simulink model "BLDCmotor_controll"  (R2015b)
settings: Solver=VariableStepAuto  StartTime=0.0  StopTime=10.0  RelTol=1e-3
settings Model: Creator=shangwei  LastModifiedBy=root

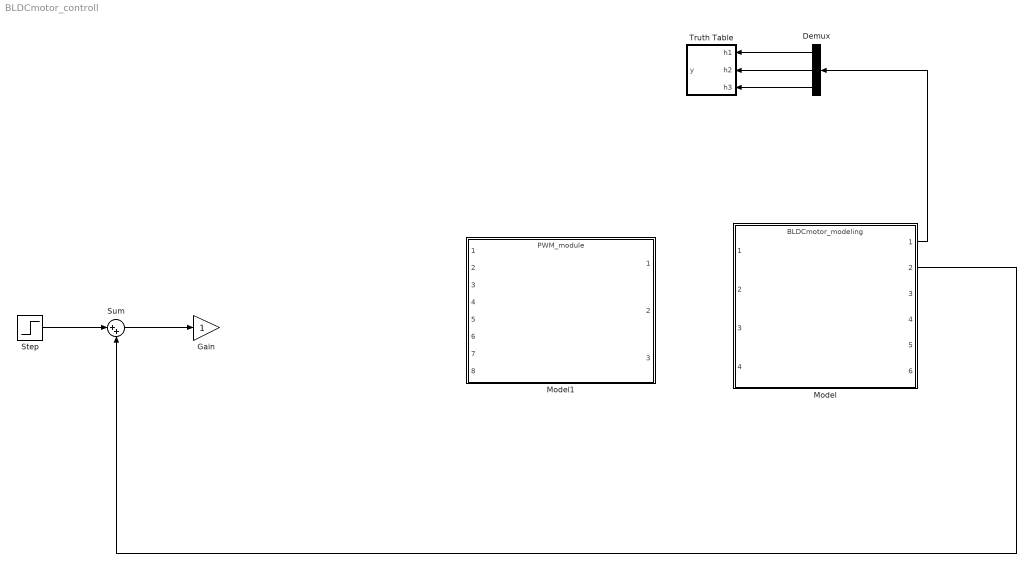
== system BLDCmotor_controll ==
  Demux : Demux  Outputs=3
  Gain : Gain
  Model : ModelReference  ModelNameDialog=BLDCmotor_modeling.slx  SimulationMode=Normal  ModelReferenceVersion=1.50  CopyOfModelName=BLDCmotor_modeling.slx
  Model1 : ModelReference  ModelNameDialog=PWM_module.slx  SimulationMode=Normal  ModelReferenceVersion=1.19  CopyOfModelName=PWM_module.slx
  Step : Step  SampleTime=0
  Sum : Sum  Inputs=|++
  Truth Table : Truth Table  TreatAsAtomicUnit=on
  wires:
  Model/2 -> Sum/2
  Step/1 -> Sum/1
  Sum/1 -> Gain/1
  Demux/2 -> Truth Table/2(h2)
  Demux/1 -> Truth Table/1(h1)
  Demux/3 -> Truth Table/3(h3)
  Model/1 -> Demux/1

== matlab function BLDCmotor_controll/Truth Table ==
  data: h1 input; y output; h2 input double; h3 input double
function y = fcn(h1, h2, h3)

aVarTruthTableCondition_1 = false;
aVarTruthTableCondition_2 = false;


% Example condition 1

aVarTruthTableCondition_1 = logical(u >= 0);

% Example condition 2

aVarTruthTableCondition_2 = logical(u ^ 2 <= 1);

if (aVarTruthTableCondition_1 && aVarTruthTableCondition_2)
    aFcnTruthTableAction_1();
elseif (~aVarTruthTableCondition_1 && ~aVarTruthTableCondition_2)
    aFcnTruthTableAction_1();
else % Default
    aFcnTruthTableAction_2();
end

function aFcnTruthTableAction_1()

% Example action 1 called from D1 & D2 column in condition table

y = u;

function aFcnTruthTableAction_2()

% Example action 2 called from D3 column in condition table

y = 1 / u;
